simulink model "aula2"  (Simulink 5.0)
settings: Solver=ode45  StartTime=0.0  StopTime=10.0  RelTol=1e-3
libraries: fuzblock x2
settings Model: BlockReductionOpt=off  BooleanDataType=off  RTWSystemTargetFile=accel.tlc  RTWTemplateMakefile=accel_default_tmf  RTWOptions="-aEnforceIntegerDowncast=1 -aFoldNonRolledExpr=1 -aForceParamTrailComments=0 -aGenerateComments=1 -aGenerateReport=0 -aIncDataTypeInIds=0 -aIncHierarchyInIds=0 -aInlineInvariantSignals=1 -aInlineParameters=0 -aInlinedPrmAccess=\"Literals\" -aLocalBlockOutputs=1 -aMaxRTWIdLen=31 -aPrefixModelToSubsysFcnNames=1 -aRTWVerbose=1 -aRollThreshold=5 -aShowEliminatedStatements=0"

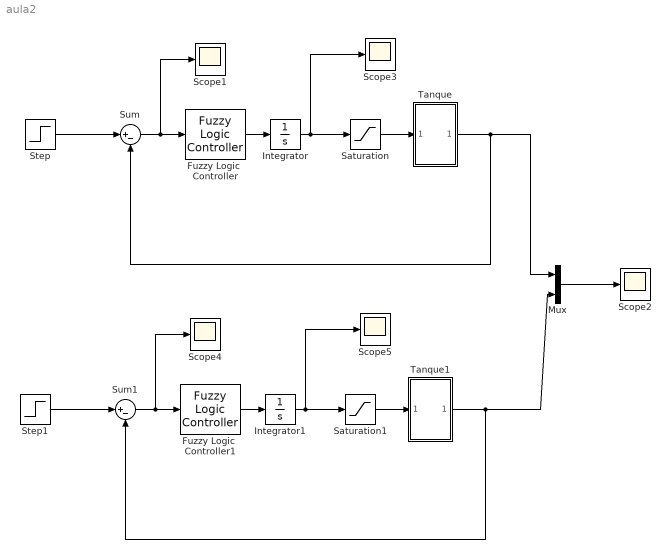
== system aula2 ==
  Fuzzy Logic  Controller : fuzblock/Fuzzy Logic  Controller  fis=aula02
  Fuzzy Logic  Controller1 : fuzblock/Fuzzy Logic  Controller  fis=aula01
  Integrator : Integrator
  Integrator1 : Integrator
  Mux : Mux  Inputs=2
  Saturation : Saturate  UpperLimit=10  LowerLimit=0
  Saturation1 : Saturate  UpperLimit=10  LowerLimit=0
  Scope{1..5} (5 alike) : Scope
      Scope3 settings: SaveName=ScopeData3
      Scope4 settings: SaveName=ScopeData4
      Scope5 settings: SaveName=ScopeData5
  Step : Step  SampleTime=0
  Step1 : Step  SampleTime=0
  Sum : Sum  Inputs=|+-  SaturateOnIntegerOverflow=on  InputSameDT=on
  Sum1 : Sum  Inputs=|+-  SaturateOnIntegerOverflow=on  InputSameDT=on
  Tanque : Subsystem
  Tanque1 : Subsystem
  wires:
  Step/1 -> Sum/1
  Sum/1 -> Fuzzy Logic  Controller/1, Scope1/1
  Fuzzy Logic  Controller/1 -> Integrator/1
  Integrator/1 -> Scope3/1, Saturation/1
  Saturation/1 -> Tanque/1(In1)
  Tanque/1(Out1) -> Sum/2, Mux/1
  Step1/1 -> Sum1/1
  Sum1/1 -> Scope4/1, Fuzzy Logic  Controller1/1
  Fuzzy Logic  Controller1/1 -> Integrator1/1
  Integrator1/1 -> Saturation1/1, Scope5/1
  Saturation1/1 -> Tanque1/1(In1)
  Tanque1/1(Out1) -> Sum1/2, Mux/2
  Mux/1 -> Scope2/1

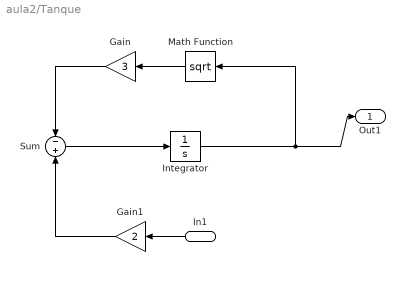
== system aula2/Tanque ==
  In1 : Inport  Orientation=left
  Gain : Gain  Orientation=left  Gain=3  SaturateOnIntegerOverflow=on
  Gain1 : Gain  Orientation=left  Gain=2  SaturateOnIntegerOverflow=on
  Integrator : Integrator  LimitOutput=on  UpperSaturationLimit=10  LowerSaturationLimit=0
  Math Function : Math  Orientation=left  Operator=sqrt  OutputSignalType=real
  Sum : Sum  Inputs=-|+  SaturateOnIntegerOverflow=on  InputSameDT=on
  Out1 : Outport
  wires:
  In1/1 -> Gain1/1
  Gain1/1 -> Sum/2
  Math Function/1 -> Gain/1
  Sum/1 -> Integrator/1
  Gain/1 -> Sum/1
  Integrator/1 -> Out1/1, Math Function/1

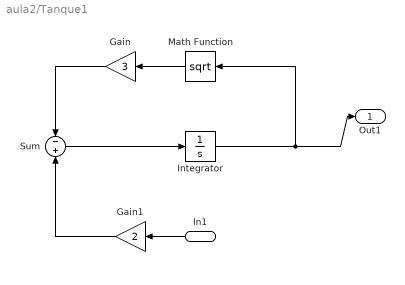
== system aula2/Tanque1 ==
  In1 : Inport  Orientation=left
  Gain : Gain  Orientation=left  Gain=3  SaturateOnIntegerOverflow=on
  Gain1 : Gain  Orientation=left  Gain=2  SaturateOnIntegerOverflow=on
  Integrator : Integrator  LimitOutput=on  UpperSaturationLimit=10  LowerSaturationLimit=0
  Math Function : Math  Orientation=left  Operator=sqrt  OutputSignalType=real
  Sum : Sum  Inputs=-|+  SaturateOnIntegerOverflow=on  InputSameDT=on
  Out1 : Outport
  wires:
  Integrator/1 -> Math Function/1, Out1/1
  Gain/1 -> Sum/1
  Sum/1 -> Integrator/1
  Math Function/1 -> Gain/1
  Gain1/1 -> Sum/2
  In1/1 -> Gain1/1
